simulink model "soc_rfsoc_top"  (R2025b)
settings: Solver=VariableStepAuto  StartTime=0.0  StopTime=4e-3  RelTol=1e-3  EnableMultiTasking=on
PreLoadFcn:
  | FrameSize = 2048;
  | NumBuffers = 16;
  | downSamplingFactor = 64;
  | SrcSel = 0;
PostLoadFcn:
  | soc_rfsoc_init(bdroot);
InitFcn:
  | soc_rfsoc_init(bdroot);
model workspace (MAT data in the model file):
  mmap = soc.memmap.MemoryMap
  mmap.isMapValid = 1
  mmap.controllerInfo = soc.memmap.MemController
  mmap.controllerInfo.memPSRange = {'2', 'G'}
  mmap.controllerInfo.memPLRange = {'2', 'G'}
  mmap.controllerInfo.memPLBaseAddrMMU = {9, '0'}
  mmap.controllerInfo.regBaseAddr = '0xA0000000'
  mmap.controllerInfo.regAddrRange = {'256', 'M'}
  mmap.map(1) = soc.memmap.MapParams
  mmap.map(1).type = 'PS Memory Region'
  mmap.map(1).name = 'AXI4-Stream to Software'
  mmap.map(1).baseAddr = '0x00000000'
  mmap.map(1).range = {'256', 'K'}
  mmap.map(1).path = 'soc_rfsoc_top/AXI4-Stream to Software'
  mmap.map(2) = soc.memmap.MapParams
  mmap.map(2).type = 'User Component'
  mmap.map(2).name = 'FPGA Tx-Rx Alg Wrapper'
  mmap.map(2).baseAddr = '0xA0000000'
  mmap.map(2).range = {'64', 'K'}
  mmap.map(2).path = 'soc_rfsoc_fpga/FPGA Tx-Rx Alg Wrapper'
  mmap.map(2).regs(1) = soc.memmap.IPCoreRegParams
  mmap.map(2).regs(1).register = 'HDL Coder registers'
  mmap.map(2).regs(1).offset = '0x0000 - 0x00FF'
  mmap.map(2).regs(1).vectorlength = 'N/A'
  mmap.map(2).regs(1).type = 'Reserved'
  mmap.map(2).regs(1).reserved = 1
  mmap.map(2).regs(2) = soc.memmap.IPCoreRegParams
  mmap.map(2).regs(2).blkname = 'FPGA Tx-Rx Alg Wrapper'
  mmap.map(2).regs(2).register = 'SrcSelReg'
  mmap.map(2).regs(2).offset = '0x0100'
  mmap.map(2).regs(2).vectorlength = '1'
  mmap.map(2).regs(2).type = 'Processor write channel'
  mmap.map(3) = soc.memmap.MapParams
  mmap.map(3).type = 'Implicit Component'
  mmap.map(3).name = 'DMAWrite'
  mmap.map(3).baseAddr = '0xA0010000'
  mmap.map(3).range = {'64', 'K'}
  mmap.map(4) = soc.memmap.MapParams
  mmap.map(4).type = 'Implicit Component'
  mmap.map(4).name = 'RFDataConverter/s_axi'
  mmap.map(4).baseAddr = '0xA3C00000'
  mmap.map(4).range = {'256', 'K'}
  mwTaskManagerKernelLatency = 0
  socvcb = containers.Map
  socvcb.serialization.keys = {157.00012207, 158.000610352, 158.000854492, 158.001220703, 158.001953125, 158.002563477, 160.001586914, 87805.0064697}
  socvcb.serialization.values : function handle (value not decoded)
  socvcb.serialization.uniformity = 0
  socvcb.serialization.keyType = 'double'
  socvcb.serialization.valueType = 'any'
undefined symbols (not defined in the file): Fs, I, m, n, Q, SampleTime
libraries: socmemlib x1, dspsrcs4 x1, proctasklib x1, xilinxrfsoclib x1
settings Model: Creator=The MathWorks, Inc.  LastModifiedBy=The MathWorks, Inc.
settings SolverCC: AlgebraicLoopSolver=TrustRegion  PositivePriorityOrder=on  AutoInsertRateTranBlk=on  MaxZcPerStep=1.0
settings DataIOCC: SaveFormat=StructureWithTime  ReturnWorkspaceOutputs=off
settings OptimizationCC: PassReuseOutputArgsAs=Individual arguments  MaxStackSize=64  EfficientTunableParamExpr=on
settings DebuggingCC: ParameterTunabilityLossMsg=error  UnconnectedInputMsg=warning  UnconnectedOutputMsg=warning  UnconnectedLineMsg=warning  ArithmeticOperatorsInVariantConditions=warning
settings HardwareCC: ProdBitPerLong=64.0  ProdLargestAtomicInteger=LongLong  ProdLargestAtomicFloat=Double  ProdLongLongMode=on  ProdHWDeviceType=ARM Compatible->ARM Cortex-A (64-bit)  HardwareBoardFeatureSet=SoCBlockset
settings ModelReferenceCC: EnableRefExpFcnMdlSchedulingChecks=on
settings SFSimCC: SimUseLocalCustomCode=off  CustomCodeUndefinedFunction=UseInterfaceOnly
settings RTWCC: SystemTargetFile=ert.tlc  HardwareBoard=Xilinx Zynq UltraScale+ RFSoC ZCU111 Evaluation Kit  TLCOptions="-aInlineSetEventsForThisBaseRateFcn=TLC_FALSE -aSuppressMultiTaskScheduler=TLC_FALSE  -aRateBasedStepFcn=0"  TemplateMakefile=ert_default_tmf  GenerateReport=on  RTWUseLocalCustomCode=off  Toolchain=Linaro AArch64 Linux v6.3.1  IncludeHyperlinkInReport=on  LaunchReport=on  GenerateTraceInfo=on  GenerateTraceReport=on  GenerateTraceReportSl=on  GenerateTraceReportSf=on  GenerateTraceReportEml=on  GPUComputeCapability=3.5  DLArmComputeVersion=19.05  Description=Embedded Coder
settings CodeAppCC: ForceParamTrailComments=on  IgnoreCustomStorageClasses=off  OperatorAnnotations=on  SimulinkDataObjDesc=on  SFDataObjDesc=on  InsertBlockDesc=on
settings ERTTargetCC: InlinedParameterPlacement=Hierarchical  DynamicArrayContainerType=coder::array

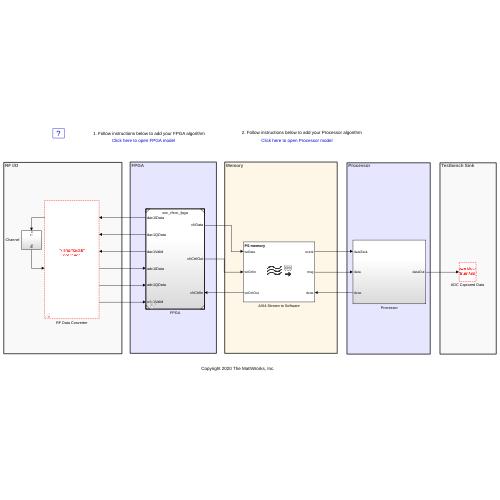
[thumbnail: Simulink's stored preview of the top-level diagram]
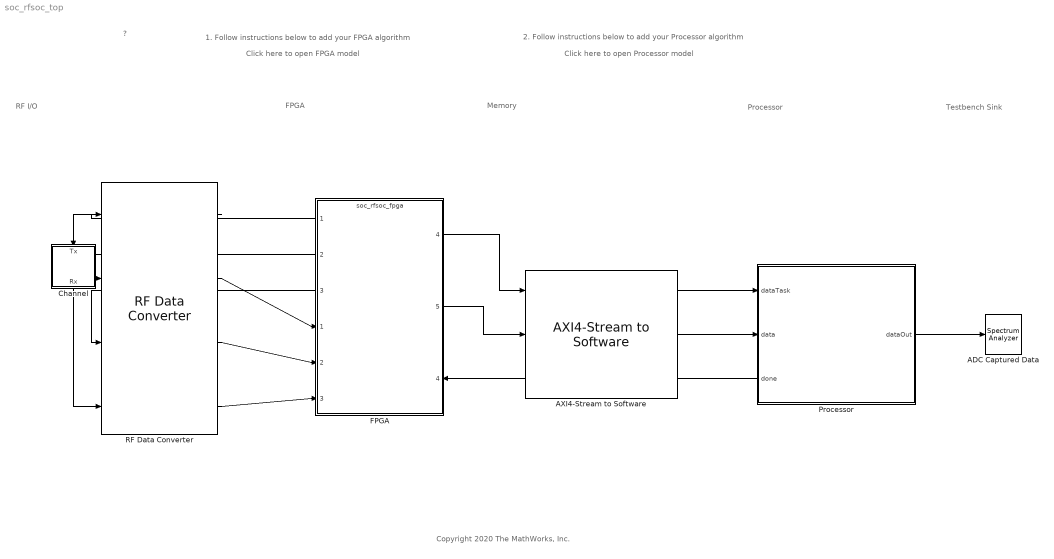
== system soc_rfsoc_top ==
  note: Click here to open FPGA model
  note: RF I/O
  note: Copyright 2020 The MathWorks, Inc.
  note: Memory
  note: Processor
  note: FPGA
  note: Testbench Sink
  note: ?
  note: 1. Follow instructions below to add your FPGA algorithm
  note: 2. Follow instructions below to add your Processor algorithm
  note: Click here to open Processor model
  ADC Captured Data : SpectrumAnalyzer  WindowPosition=[560.000000,350.000000,800.000000,500.000000,]  ScopeFrameLocation=window  WindowInvariantSamplesPerUpdate=on  YLimits=[8.5344 101.7178]  SelectedToolstripTab=spectrumAnalyzerToolstrip.measurementsTab
  AXI4-Stream to Software : socmemlib/AXI4-Stream to Software  MemorySimulation=Burst accurate  MemorySelection=PS memory  MRNumBuffers=NumBuffers  BurstLengthWriterChIf=256  FIFODepthWriter=8  FIFOAFullDepthWriter=6  ICClockFrequencyWriter=300  ICDataWidthWriter=64  ChDimensionsWriterChIf=1  ChTypeWriterChIf=uint64  ChFrameSampleTimeWriterChIf=SampleTime  ChBitPackedWriterChIf=off  ChDimensionsReaderChIf=FrameSize  ChTypeReaderChIf=uint64  LastTargetBoard=Xilinx Zynq UltraScale+ RFSoC ZCU111 Evaluation Kit  MRRegionSize=262144  MRBufferSize=16384  DiagnosticLevel=Basic diagnostic signals
  Channel : Subsystem
  FPGA : ModelReference  ModelNameDialog=soc_rfsoc_fpga.slx  SimulationMode=Normal  ModelReferenceVersion=9.0
      settings: PortSchema="{\"entries\":[{\"content\":{\"sides\":[{\"content\":{\"connectorIds\":[\"Out1\",\"Out2\",\"Out3\",\"In1\",\"In2\",\"In3\"]},\"type\":\"ConnectorPlacement.EquallySpacedRectSide\",\"uuid\":\"5cb1a72a-01db-451a-a1d5-13c90475b746\"},{\"content\":{\"connectorIds\":[\"Out4\",\"Out5\",\"In4\"],\"side\":\"RIGHT\"},\"type\":\"ConnectorPlacement.EquallySpacedRectSide\",\"uuid\":\"0cc5c425-085f-4d55-8809-74a02be1a373\"},{\"content\":{\"connectorIds\":[],\"side\":\"TOP\"},\"type\":\"ConnectorPlacement.EquallySpacedRectSide\",\"uuid\":\"74405138-49c7-488d-8705-1658c6d2c17e\"},{\"content\":{\"connectorIds\":[],\"side\":\"BOTTOM\"},\"type\":\"ConnectorPlacement.EquallySpacedRectSide\",\"uuid\":\"41d3b708-b00f-42a5-bfad-1616ef33dc5f\"}]},\"type\":\"ConnectorPlacement.EquallySpacedConnector\",\"uuid\":\"fa285e06-79f7-4ad6-b6b8-2363bd8486be\"}],\"packageUris\":[\"http://schema.mathworks.com/mf0/Connector/19700101\"],\"version\":\"1.0\"}"
  Processor : Subsystem
      settings: PortSchema="{\"entries\":[{\"content\":{\"sides\":[{\"content\":{\"connectorIds\":[\"In1\",\"In2\",\"Out2\"]},\"type\":\"ConnectorPlacement.EquallySpacedRectSide\",\"uuid\":\"c6517cf8-029b-42a5-8e0a-4a74babda661\"},{\"content\":{\"connectorIds\":[\"Out1\"],\"side\":\"RIGHT\"},\"type\":\"ConnectorPlacement.EquallySpacedRectSide\",\"uuid\":\"16c669d3-b531-49c5-97c0-aad9de53fc76\"},{\"content\":{\"connectorIds\":[],\"side\":\"TOP\"},\"type\":\"ConnectorPlacement.EquallySpacedRectSide\",\"uuid\":\"ee928f87-c942-476b-86c6-8f97cdee9f2e\"},{\"content\":{\"connectorIds\":[],\"side\":\"BOTTOM\"},\"type\":\"ConnectorPlacement.EquallySpacedRectSide\",\"uuid\":\"ef0c39df-7d54-4afb-ba81-784fc61f5805\"}]},\"type\":\"ConnectorPlacement.EquallySpacedConnector\",\"uuid\":\"c956b2ab-b210-4cbd-a6ac-ba45bfad9e74\"}],\"packageUris\":[\"http://schema.mathworks.com/mf0/Connector/19700101\"],\"version\":\"1.0\"}"
  RF Data Converter : xilinxrfsoclib/RF Data Converter  RFDCSim=Behavioral  tabPromptsCB=0  RFInterface=Customize  digitalInterface=I/Q  dac11Enable=off  dac12Enable=off  dac13Enable=off  dac14Enable=off  dac21Enable=off  dac22Enable=off  dac23Enable=on  dac24Enable=off  dac31Enable=off  dac32Enable=off  dac33Enable=off  dac34Enable=off  dac41Enable=off  dac42Enable=off  dac43Enable=off  dac44Enable=off  matchDACParam=on  dacSampleRate=1024  dacDatapathMode=Full Nyquist (0 to Fs/2)  interpolationMode=4  dacSamplesPerCycle=2  dacMixerType=Fine  dacMixerMode=I/Q->Real  dacMixerFrequency=Fs/4  dacNCOFrequency=0.3  dacNCOPhase=0  invertSyncFilter=off  dacTile1SampleRate=1000  dac11DatapathMode=Full Nyquist (0 to Fs/2)  dac11InterpolationMode=2  dac11SamplesPerCycle=2  dac11MixerType=Coarse  dac11MixerMode=I/Q->Real  dac11MixerFrequency=Fs/2  dac11NCOFrequency=0  dac11NCOPhase=0  dac11InvertSyncFilter=off  dac12DatapathMode=Full Nyquist (0 to Fs/2)  dac12InterpolationMode=2  dac12SamplesPerCycle=2  dac12MixerType=Coarse  dac12MixerMode=I/Q->Real  dac12MixerFrequency=Fs/2  dac12NCOFrequency=0  dac12NCOPhase=0  dac12InvertSyncFilter=off  dac13DatapathMode=Full Nyquist (0 to Fs/2)  dac13InterpolationMode=2  dac13SamplesPerCycle=2  dac13MixerType=Coarse  dac13MixerMode=I/Q->Real  dac13MixerFrequency=Fs/2  dac13NCOFrequency=0  dac13NCOPhase=0  dac13InvertSyncFilter=off  dac14DatapathMode=Full Nyquist (0 to Fs/2)  dac14InterpolationMode=2  dac14SamplesPerCycle=2  dac14MixerType=Coarse  dac14MixerMode=I/Q->Real  dac14MixerFrequency=Fs/2  dac14NCOFrequency=0  dac14NCOPhase=0  dac14InvertSyncFilter=off  dacTile2SampleRate=1000  dac21DatapathMode=Full Nyquist (0 to Fs/2)  dac21InterpolationMode=2  dac21SamplesPerCycle=2  dac21MixerType=Coarse  dac21MixerMode=I/Q->Real  dac21MixerFrequency=Fs/2  dac21NCOFrequency=0  dac21NCOPhase=0  dac21InvertSyncFilter=off  dac22DatapathMode=Full Nyquist (0 to Fs/2)  dac22InterpolationMode=2  dac22SamplesPerCycle=2  dac22MixerType=Coarse  dac22MixerMode=I/Q->Real  dac22MixerFrequency=Fs/2  dac22NCOFrequency=0  dac22NCOPhase=0  dac22InvertSyncFilter=off  dac23DatapathMode=Full Nyquist (0 to Fs/2)  dac23InterpolationMode=2  dac23SamplesPerCycle=2  dac23MixerType=Coarse  dac23MixerMode=I/Q->Real  dac23MixerFrequency=Fs/2  dac23NCOFrequency=0  dac23NCOPhase=0  dac23InvertSyncFilter=off  dac24DatapathMode=Full Nyquist (0 to Fs/2)  dac24InterpolationMode=2  dac24SamplesPerCycle=2  dac24MixerType=Coarse  dac24MixerMode=I/Q->Real  dac24MixerFrequency=Fs/2  dac24NCOFrequency=0  dac24NCOPhase=0  dac24InvertSyncFilter=off  dacTile3SampleRate=1000  dac31DatapathMode=Full Nyquist (0 to Fs/2)  dac31InterpolationMode=2  dac31SamplesPerCycle=2  dac31MixerType=Coarse  dac31MixerMode=I/Q->Real  dac31MixerFrequency=Fs/2  dac31NCOFrequency=0  dac31NCOPhase=0  dac31InvertSyncFilter=off  dac32DatapathMode=Full Nyquist (0 to Fs/2)  dac32InterpolationMode=2  dac32SamplesPerCycle=2  dac32MixerType=Coarse  dac32MixerMode=I/Q->Real  dac32MixerFrequency=Fs/2  dac32NCOFrequency=0  dac32NCOPhase=0  dac32InvertSyncFilter=off  dac33DatapathMode=Full Nyquist (0 to Fs/2)  dac33InterpolationMode=2  dac33SamplesPerCycle=2  dac33MixerType=Coarse  dac33MixerMode=I/Q->Real  dac33MixerFrequency=Fs/2  dac33NCOFrequency=0  dac33NCOPhase=0  dac33InvertSyncFilter=off  dac34DatapathMode=Full Nyquist (0 to Fs/2)  dac34InterpolationMode=2  dac34SamplesPerCycle=2  dac34MixerType=Coarse  dac34MixerMode=I/Q->Real  dac34MixerFrequency=Fs/2  dac34NCOFrequency=0  dac34NCOPhase=0  dac34InvertSyncFilter=off  dacTile4SampleRate=1000  dac41DatapathMode=Full Nyquist (0 to Fs/2)  dac41InterpolationMode=2  dac41SamplesPerCycle=2  dac41MixerType=Coarse  dac41MixerMode=I/Q->Real  dac41MixerFrequency=Fs/2  dac41NCOFrequency=0  dac41NCOPhase=0  dac41InvertSyncFilter=off  dac42DatapathMode=Full Nyquist (0 to Fs/2)  dac42InterpolationMode=2  dac42SamplesPerCycle=2  dac42MixerType=Coarse  dac42MixerMode=I/Q->Real  dac42MixerFrequency=Fs/2  dac42NCOFrequency=0  dac42NCOPhase=0  dac42InvertSyncFilter=off  dac43DatapathMode=Full Nyquist (0 to Fs/2)  dac43InterpolationMode=2  dac43SamplesPerCycle=2  dac43MixerType=Coarse  dac43MixerMode=I/Q->Real  dac43MixerFrequency=Fs/2  dac43NCOFrequency=0  dac43NCOPhase=0  dac43InvertSyncFilter=off  dac44DatapathMode=Full Nyquist (0 to Fs/2)  dac44InterpolationMode=2  dac44SamplesPerCycle=2  dac44MixerType=Coarse  dac44MixerMode=I/Q->Real  dac44MixerFrequency=Fs/2  dac44NCOFrequency=0  dac44NCOPhase=0  dac44InvertSyncFilter=off  adc11Enable=on  adc12Enable=off  adc13Enable=off  adc14Enable=off  adc21Enable=off  adc22Enable=off  adc23Enable=off  adc24Enable=off  adc31Enable=off  adc32Enable=off  adc33Enable=off  adc34Enable=off  adc41Enable=off  adc42Enable=off  adc43Enable=off  adc44Enable=off  adcOutUnpackedData=on  matchADCParam=on  adcSampleRate=1024  decimationMode=4  adcSamplesPerCycle=2  adcMixerType=Fine  adcMixerMode=Real->I/Q  adcMixerFrequency=-Fs/4  adcNCOFrequency=-0.3  adcNCOPhase=0  adcTile1SampleRate=1000  adc11DecimationMode=2  adc11SamplesPerCycle=2  adc11MixerType=Coarse  adc11MixerMode=Real->I/Q  adc11MixerFrequency=Fs/2  adc11NCOFrequency=0  adc11NCOPhase=0  adc12DecimationMode=2  adc12SamplesPerCycle=2  adc12MixerType=Coarse  adc12MixerMode=Real->I/Q  adc12MixerFrequency=Fs/2  adc12NCOFrequency=0  adc12NCOPhase=0  adc13DecimationMode=2  adc13SamplesPerCycle=2  adc13MixerType=Coarse  adc13MixerMode=Real->I/Q  adc13MixerFrequency=Fs/2  adc13NCOFrequency=0  adc13NCOPhase=0  adc14DecimationMode=2  adc14SamplesPerCycle=2  adc14MixerType=Coarse  adc14MixerMode=Real->I/Q  adc14MixerFrequency=Fs/2  adc14NCOFrequency=0  adc14NCOPhase=0  adcTile2SampleRate=1000  adc21DecimationMode=2  adc21SamplesPerCycle=2  adc21MixerType=Coarse  adc21MixerMode=Real->I/Q  adc21MixerFrequency=Fs/2  adc21NCOFrequency=0  adc21NCOPhase=0  adc22DecimationMode=2  adc22SamplesPerCycle=2  adc22MixerType=Coarse  adc22MixerMode=Real->I/Q  adc22MixerFrequency=Fs/2  adc22NCOFrequency=0  adc22NCOPhase=0  adc23DecimationMode=2  adc23SamplesPerCycle=2  adc23MixerType=Coarse  adc23MixerMode=Real->I/Q  adc23MixerFrequency=Fs/2  adc23NCOFrequency=0  adc23NCOPhase=0  adc24DecimationMode=2  adc24SamplesPerCycle=2  adc24MixerType=Coarse  adc24MixerMode=Real->I/Q  adc24MixerFrequency=Fs/2  adc24NCOFrequency=0  adc24NCOPhase=0  adcTile3SampleRate=1000  adc31DecimationMode=2  adc31SamplesPerCycle=2  adc31MixerType=Coarse  adc31MixerMode=Real->I/Q  adc31MixerFrequency=Fs/2  adc31NCOFrequency=0  adc31NCOPhase=0  adc32DecimationMode=2  adc32SamplesPerCycle=2  adc32MixerType=Coarse  adc32MixerMode=Real->I/Q  adc32MixerFrequency=Fs/2  adc32NCOFrequency=0  adc32NCOPhase=0  adc33DecimationMode=2  adc33SamplesPerCycle=2  adc33MixerType=Coarse  adc33MixerMode=Real->I/Q  adc33MixerFrequency=Fs/2  adc33NCOFrequency=0  adc33NCOPhase=0  adc34DecimationMode=2  adc34SamplesPerCycle=2  adc34MixerType=Coarse  adc34MixerMode=Real->I/Q  adc34MixerFrequency=Fs/2  adc34NCOFrequency=0  adc34NCOPhase=0  adcTile4SampleRate=1000  adc41DecimationMode=2  adc41SamplesPerCycle=2  adc41MixerType=Coarse  adc41MixerMode=Real->I/Q  adc41MixerFrequency=Fs/2  adc41NCOFrequency=0  adc41NCOPhase=0  adc42DecimationMode=2  adc42SamplesPerCycle=2  adc42MixerType=Coarse  adc42MixerMode=Real->I/Q  adc42MixerFrequency=Fs/2  adc42NCOFrequency=0  adc42NCOPhase=0  adc43DecimationMode=2  adc43SamplesPerCycle=2  adc43MixerType=Coarse  adc43MixerMode=Real->I/Q  adc43MixerFrequency=Fs/2  adc43NCOFrequency=0  adc43NCOPhase=0  adc44DecimationMode=2  adc44SamplesPerCycle=2  adc44MixerType=Coarse  adc44MixerMode=Real->I/Q  adc44MixerFrequency=Fs/2  adc44NCOFrequency=0  adc44NCOPhase=0  multiTileSync=off  externalPLL=off  dacRealTimeNCOPortsEnable=off  adcRealTimeNCOPortsEnable=off  adcRealTimePortsEnable=off  adcThresholdMode=Sticky over  adcThreshold1=0  adcDelayCounter=0  adcThreshold2Mode=Sticky over  adcThreshold2=0  adcThreshold2DelayCounter=0  adc11ThresholdMode=Sticky over  adc11Threshold1=0  adc11DelayCounter=0  adc11Threshold2Mode=Sticky over  adc11Threshold2=0  adc11Threshold2DelayCounter=0  adc12ThresholdMode=Sticky over  adc12Threshold1=0  adc12DelayCounter=0  adc12Threshold2Mode=Sticky over  adc12Threshold2=0  adc12Threshold2DelayCounter=0  adc13ThresholdMode=Sticky over  adc13Threshold1=0  adc13DelayCounter=0  adc13Threshold2Mode=Sticky over  adc13Threshold2=0  adc13Threshold2DelayCounter=0  adc14ThresholdMode=Sticky over  adc14Threshold1=0  adc14DelayCounter=0  adc14Threshold2Mode=Sticky over  adc14Threshold2=0  adc14Threshold2DelayCounter=0  adc21ThresholdMode=Sticky over  adc21Threshold1=0  adc21DelayCounter=0  adc21Threshold2Mode=Sticky over  adc21Threshold2=0  adc21Threshold2DelayCounter=0  adc22ThresholdMode=Sticky over  adc22Threshold1=0  adc22DelayCounter=0  adc22Threshold2Mode=Sticky over  adc22Threshold2=0  adc22Threshold2DelayCounter=0  adc23ThresholdMode=Sticky over  adc23Threshold1=0  adc23DelayCounter=0  adc23Threshold2Mode=Sticky over  adc23Threshold2=0  adc23Threshold2DelayCounter=0  adc24ThresholdMode=Sticky over  adc24Threshold1=0  adc24DelayCounter=0  adc24Threshold2Mode=Sticky over  adc24Threshold2=0  adc24Threshold2DelayCounter=0  adc31ThresholdMode=Sticky over  adc31Threshold1=0  adc31DelayCounter=0  adc31Threshold2Mode=Sticky over  adc31Threshold2=0  adc31Threshold2DelayCounter=0  adc32ThresholdMode=Sticky over  adc32Threshold1=0  adc32DelayCounter=0  adc32Threshold2Mode=Sticky over  adc32Threshold2=0  adc32Threshold2DelayCounter=0  adc33ThresholdMode=Sticky over  adc33Threshold1=0  adc33DelayCounter=0  adc33Threshold2Mode=Sticky over  adc33Threshold2=0  adc33Threshold2DelayCounter=0  adc34ThresholdMode=Sticky over  adc34Threshold1=0  adc34DelayCounter=0  adc34Threshold2Mode=Sticky over  adc34Threshold2=0  adc34Threshold2DelayCounter=0  adc41ThresholdMode=Sticky over  adc41Threshold1=0  adc41DelayCounter=0  adc41Threshold2Mode=Sticky over  adc41Threshold2=0  adc41Threshold2DelayCounter=0  adc42ThresholdMode=Sticky over  adc42Threshold1=0  adc42DelayCounter=0  adc42Threshold2Mode=Sticky over  adc42Threshold2=0  adc42Threshold2DelayCounter=0  adc43ThresholdMode=Sticky over  adc43Threshold1=0  adc43DelayCounter=0  adc43Threshold2Mode=Sticky over  adc43Threshold2=0  adc43Threshold2DelayCounter=0  adc44ThresholdMode=Sticky over  adc44Threshold1=0  adc44DelayCounter=0  adc44Threshold2Mode=Sticky over  adc44Threshold2=0  adc44Threshold2DelayCounter=0
  wires:
  RF Data Converter/1 -> Channel/1(Tx)
  Processor/1(dataOut) -> ADC Captured Data/1
  FPGA/4 -> AXI4-Stream to Software/1
  FPGA/5 -> AXI4-Stream to Software/2
  AXI4-Stream to Software/1 -> Processor/1(dataTask)
  AXI4-Stream to Software/2 -> Processor/2(data)
  Processor/2(done) -> AXI4-Stream to Software/3
  RF Data Converter/2 -> FPGA/1
  Channel/1(Rx) -> RF Data Converter/4
  RF Data Converter/3 -> FPGA/2
  RF Data Converter/4 -> FPGA/3
  AXI4-Stream to Software/3 -> FPGA/4
  FPGA/1 -> RF Data Converter/1
  FPGA/2 -> RF Data Converter/2
  FPGA/3 -> RF Data Converter/3

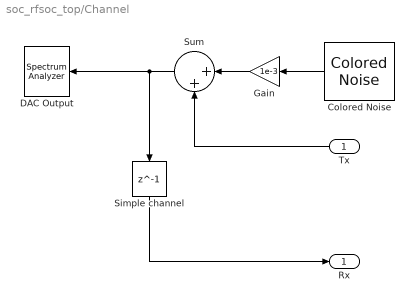
== system soc_rfsoc_top/Channel ==
  Tx : Inport
  Colored Noise : dspsrcs4/Colored Noise  Color=white  InverseFrequencyPower=1  BoundedOutput=off  NumChannels=1  OutputDataType=double  SamplesPerFrame=4*2  SampleTime=1/1024e6  RandomStream=mt19937ar with seed  Seed=67  SimulateUsing=Interpreted execution
  DAC Output : SpectrumAnalyzer  WindowPosition=[560.000000,350.000000,800.000000,500.000000,]  ScopeFrameLocation=window  PlotAsTwoSidedSpectrum=off  WindowInvariantSamplesPerUpdate=on  YLimits=[-73.4396 24.4214]  SelectedToolstripTab=spectrumAnalyzerToolstrip.spectrumTab
  Gain : Gain  Gain=1e-3  OutDataTypeStr=double
  Simple channel : Delay  DelayLength=1
  Sum : Sum  Inputs=|++
  Rx : Outport  VectorParamsAs1DForOutWhenUnconnected=off
  wires:
  Simple channel/1 -> Rx/1
  Colored Noise/1 -> Gain/1
  Gain/1 -> Sum/1
  Tx/1 -> Sum/2
  Sum/1 -> DAC Output/1, Simple channel/1

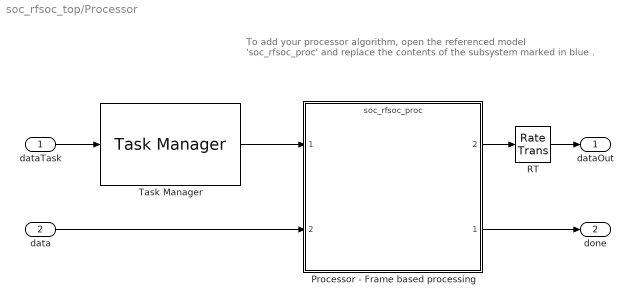
== system soc_rfsoc_top/Processor ==
  note: To add your processor algorithm, open the referenced model 'soc_rfsoc_proc' and replace the contents of the subsystem marked in blue .
  dataTask : Inport
  data : Inport  Port=2
  Processor - Frame based processing : ModelReference  InputPortMessageModes=n,m  OutputPortMessageModes=m,n  ModelNameDialog=soc_rfsoc_proc.slx  SimulationMode=Normal  ModelReferenceVersion=3.2
      settings: PortSchema="{\"entries\":[{\"content\":{\"sides\":[{\"content\":{\"connectorIds\":[\"In1\",\"In2\"]},\"type\":\"ConnectorPlacement.EquallySpacedRectSide\",\"uuid\":\"9bed6bab-e1e2-4bbd-ad7b-1faa1b6c1798\"},{\"content\":{\"connectorIds\":[\"Out2\",\"Out1\"],\"side\":\"RIGHT\"},\"type\":\"ConnectorPlacement.EquallySpacedRectSide\",\"uuid\":\"81dc2d70-e9c6-4efe-b2f0-f510dafcf226\"},{\"content\":{\"connectorIds\":[],\"side\":\"TOP\"},\"type\":\"ConnectorPlacement.EquallySpacedRectSide\",\"uuid\":\"bcde9838-fab9-4316-8c6c-5e2bf6cf8acb\"}]},\"type\":\"ConnectorPlacement.EquallySpacedConnector\",\"uuid\":\"60a6370a-2c5c-4560-bd50-f52abe546349\"}],\"packageUris\":[\"http://schema.mathworks.com/mf0/Connector/19700101\"],\"version\":\"1.0\"}"
  RT : RateTransition  Integrity=off  Deterministic=off  OutPortSampleTime=FrameSize*SampleTime*downSamplingFactor
  Task Manager : proctasklib/Task Manager  AllTaskData="{\"taskName\":\"DataReadTask\",\"taskType\":\"Event-driven\",\"taskEvent\":\"DataReadTaskEvent\",\"taskPeriod\":\"0.1\",\"taskPriority\":\"50\",\"coreSelection\":\"Specified core\",\"coreNum\":\"0\",\"dropOverranTasks\":false,\"playbackRecorded\":false,\"diagnosticsFile\":\"\",\"taskDurationSource\":\"Dialog\",\"taskDuration\":0.000101031,\"taskDurationDeviation\":1.3727E-5,\"logExecutionData\":true,\"logDroppedTasks\":false,\"version\":\"2.6\",\"taskDurationData\":{\"percent\":[\"100\"],\"mean\":[\"0.5e-3\"],\"dev\":[\"0\"],\"min\":[\"0.5e-3\"],\"max\":[\"0.5e-3\"]},\"taskEventSource\":\"AXI4-Stream to Software\",\"taskEventSourceAssignmentType\":\"AutoAssigned\",\"taskEventSourceType\":\"Stream\",\"taskEventGroup\":\"Unspecified\",\"taskEventInterrupt\":\"Unspecified\",\"taskEventOrder\":1,\"taskDisablePremption\":false,\"taskClearInterruptFlagsAtEndOfEvent\":false}"  EnableTaskSimulation=on  StreamToSDI=on  WriteToFile=off  OverwriteFile=off  SupportEventPorts=on  UseScheduleEditor=off  CustomizationInfo=''
  dataOut : Outport  VectorParamsAs1DForOutWhenUnconnected=off
  done : Outport  Port=2  VectorParamsAs1DForOutWhenUnconnected=off
  wires:
  data/1 -> Processor - Frame based processing/2
  dataTask/1 -> Task Manager/1
  Task Manager/1 -> Processor - Frame based processing/1
  Processor - Frame based processing/2 -> RT/1
  Processor - Frame based processing/1 -> done/1
  RT/1 -> dataOut/1
